simulink model "Current_reversible_chopper"  (Simulink 7.9)
settings: Solver=ode23tb  StartTime=0.0  StopTime=0.03  MaxStep=2e-5  RelTol=1e-3  AbsTol=.1
libraries: powerlib x8
settings Model: Creator=lanyi  LastModifiedBy=lanyi
settings OptimizationCC: InlineInvariantSignals=on  InitFltsAndDblsToZero=on
settings DebuggingCC: SaveWithParameterizedLinksMsg=none  SignalResolutionControl=TryResolveAllWithWarning  MultiTaskDSMMsg=warning  MultiTaskCondExecSysMsg=none  FcnCallInpInsideContextMsg=Use local settings  StrictBusMsg=None
settings RTWCC: IncludeERTFirstTime=on
settings GRTTargetCC: TargetFcnLib=ansi_tfl_tmw.mat  CombineOutputUpdateFcns=off  GRTInterface=on

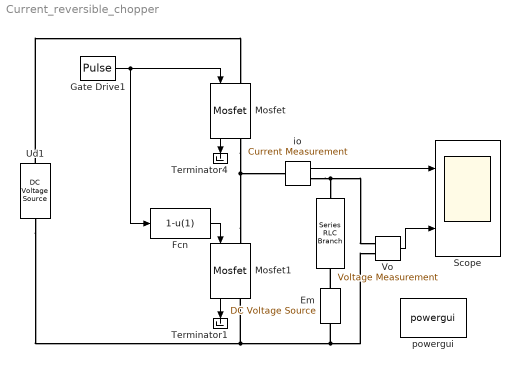
== system Current_reversible_chopper ==
  " " : powerlib/Elements/Series RLC Branch  LConnTagsString=__new0  RConnTagsString=__new0  BranchType=RL  Resistance=1  Inductance=0.001  SetiL0=off  InitialCurrent=0  Capacitance=inf  Setx0=off  InitialVoltage=0  Measurements=None
  Em : powerlib/Electrical Sources/DC Voltage Source  Amplitude=50  Measurements=None
  Fcn : Fcn  Expr=1-u(1)
  Gate Drive1 : DiscretePulseGenerator  PulseType=Time based  Period=0.001  PulseWidth=70
  Mosfet : powerlib/Power Electronics/Mosfet  Ron=0.001  Lon=1e-9  Rd=.001  Vfd=0  IC=0  Rs=1  Cs=1e-6  Measurements=on
  Mosfet1 : powerlib/Power Electronics/Mosfet  Ron=0.001  Lon=1e-9  Rd=.001  Vfd=0  IC=0  Rs=1  Cs=1e-6  Measurements=on
  Scope : Scope  NumInputPorts=2
      settings: TimeRange=0.01  YMin=-100~-50  YMax=100~150  SampleTime=2e-4
  Terminator1 : Terminator
  Terminator4 : Terminator
  Ud1 : powerlib/Electrical Sources/DC Voltage Source  Amplitude=100  Measurements=None
  Vo : powerlib/Measurements/Voltage Measurement  PhasorSimulation=off  OutputType=Complex  PSBequivalent=0
  io : powerlib/Measurements/Current Measurement  PhasorSimulation=off  OutputType=Complex  PSBequivalent=0
  powergui : powerlib/powergui  Priority=1  SimulationMode=Continuous  SolverType=Tustin  SampleTime=50e-6  frequency=60  SPID=off  DisableSnubberDevices=off  DisableRonSwitches=off  DisableVfSwitches=off  SwTol=0  Interpol=off  DisplayEquations=off  FunctionMessages=off  frequencyindice=0  Pbase=100e6  ErrMax=1e-4  Iterations=50  UnitsV=kV  UnitsW=MW  echomessages=off  HookPort=off  EnableUseOfTLC=off  x0status=blocks  RestoreLinks=warning  ResistiveCurrentMeasurement=off  Ylog=off  Xlog=on  ShowGrid=off  save=off  variable=ZData  ZoomFFT=off  StartTime=0.0  cycles=1  DisplayStyle=1  FreqAxis=off  MaxFrequency=1000  frequencyindicesteady=1  display=off  methode=off
  wires:
  Vo/1 -> Scope/2
  Fcn/1 -> Mosfet1/1
  Gate Drive1/1 -> Fcn/1, Mosfet/1
  io/1 -> Scope/1
  Mosfet/1 -> Terminator4/1
  Mosfet1/1 -> Terminator1/1
  connections:
  Mosfet1/RConn1 -- Em/LConn1 -- Vo/LConn2 -- Ud1/LConn1
  Mosfet1/LConn1 -- io/LConn1 -- Mosfet/RConn1
  Ud1/RConn1 -- Mosfet/LConn1
  io/RConn1 -- " "/LConn1 -- Vo/LConn1
  Em/RConn1 -- " "/RConn1
